simulink model "shape_nowlin"  (R2020b)
settings: Solver=VariableStepAuto  StartTime=0.0  StopTime=10.0  RelTol=1e-3
model workspace (MAT data in the model file):
  f_attenuation = Simulink.Parameter
  f_attenuation.Value = 0.5
  f_attenuation.DataType = 'double'
  f_attenuation.Dimensions = [1 1]
libraries: simulink x1
settings Model: ParameterArgumentNames=f_attenuation  OrderedModelArguments=off  Creator=lydialee  LastModifiedBy=lydialee
settings SFSimCC: CustomCodeUndefinedFunction=UseInterfaceOnly

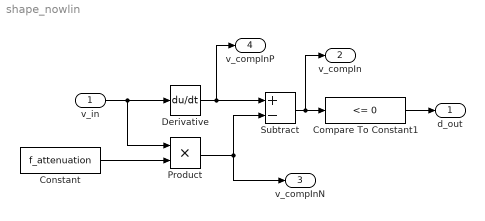
== system shape_nowlin ==
  v_in : Inport
  Compare To Constant1 : simulink/Logic and Bit Operations/Compare To Constant  relop=<=  const=0  OutDataTypeStr=boolean
  Constant : Constant  Value=f_attenuation
  Derivative : Derivative
  Product : Product
  Subtract : Sum  Inputs=+-
  d_out : Outport  VectorParamsAs1DForOutWhenUnconnected=off
  v_compIn : Outport  Port=2  VectorParamsAs1DForOutWhenUnconnected=off
  v_compInN : Outport  Port=3  VectorParamsAs1DForOutWhenUnconnected=off
  v_compInP : Outport  Port=4  VectorParamsAs1DForOutWhenUnconnected=off
  wires:
  Compare To Constant1/1 -> d_out/1
  Subtract/1 -> v_compIn/1, Compare To Constant1/1
  v_in/1 -> Product/1, Derivative/1
  Derivative/1 -> v_compInP/1, Subtract/1
  Product/1 -> v_compInN/1, Subtract/2
  Constant/1 -> Product/2
